simulink model "yorkFromSimu"  (Simulink 7.2)
settings: Solver=ode45  StartTime=0.0  StopTime=10.0  RelTol=1e-3
settings Model: Creator=alesch  LastModifiedBy=alesch

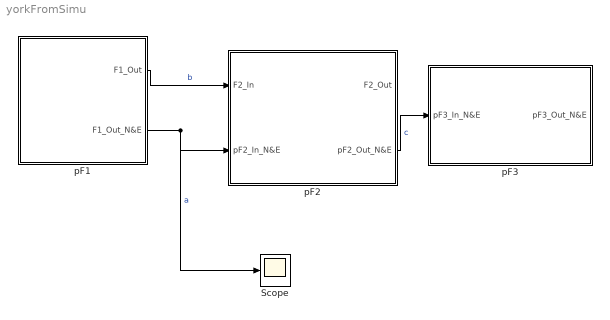
== system yorkFromSimu ==
  Scope : Scope
  pF1 : Subsystem
  pF2 : Subsystem
  pF3 : Subsystem
  wires:
  pF1/1(F1_Out) -> pF2/1(F2_In)  "b"
  pF2/2(pF2_Out_N&E) -> pF3/1(pF3_In_N&E)  "c"
  pF1/2(F1_Out_N&E) -> Scope/1, pF2/2(pF2_In_N&E)  "a"

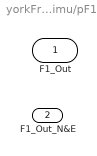
== system yorkFromSimu/pF1 ==
  F1_Out : Outport  OutDataType=sfix(16)  OutScaling=2^0
  F1_Out_N&E : Outport  Port=2  OutDataType=sfix(16)  OutScaling=2^0

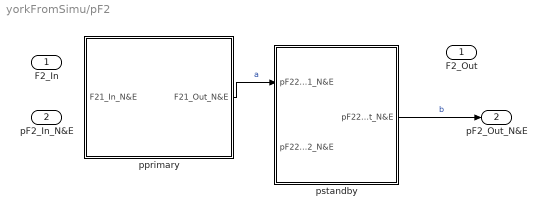
== system yorkFromSimu/pF2 ==
  F2_In : Inport  OutDataType=sfix(16)  OutScaling=2^0
  pF2_In_N&E : Inport  Port=2  OutDataType=sfix(16)  OutScaling=2^0
  pprimary : Subsystem
  pstandby : Subsystem
  F2_Out : Outport  OutDataType=sfix(16)  OutScaling=2^0
  pF2_Out_N&E : Outport  Port=2  OutDataType=sfix(16)  OutScaling=2^0
  wires:
  pprimary/1(F21_Out_N&E) -> pstandby/1(pF22_In1_N&E)  "a"
  pstandby/1(pF22_Out_N&E) -> pF2_Out_N&E/1  "b"

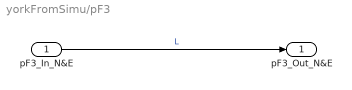
== system yorkFromSimu/pF3 ==
  pF3_In_N&E : Inport  OutDataType=sfix(16)  OutScaling=2^0
  pF3_Out_N&E : Outport  OutDataType=sfix(16)  OutScaling=2^0
  wires:
  pF3_In_N&E/1 -> pF3_Out_N&E/1  "L"

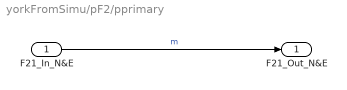
== system yorkFromSimu/pF2/pprimary ==
  F21_In_N&E : Inport  OutDataType=sfix(16)  OutScaling=2^0
  F21_Out_N&E : Outport  OutDataType=sfix(16)  OutScaling=2^0
  wires:
  F21_In_N&E/1 -> F21_Out_N&E/1  "m"

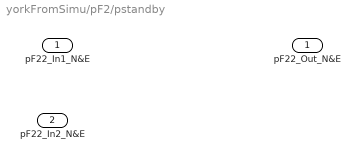
== system yorkFromSimu/pF2/pstandby ==
  pF22_In1_N&E : Inport  OutDataType=sfix(16)  OutScaling=2^0
  pF22_In2_N&E : Inport  Port=2  OutDataType=sfix(16)  OutScaling=2^0
  pF22_Out_N&E : Outport  OutDataType=sfix(16)  OutScaling=2^0
